simulink model "IQRD_RLS_model_top_3x3"  (R2020b)
settings: Solver=VariableStepAuto  StartTime=0.0  StopTime=0.00001  RelTol=1e-3
settings Model: Creator=jgentile  LastModifiedBy=jgentile

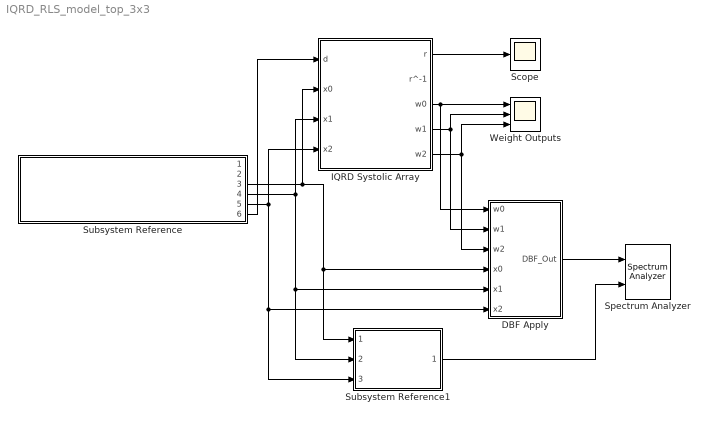
== system IQRD_RLS_model_top_3x3 ==
  DBF Apply : Subsystem
  IQRD Systolic Array : Subsystem
  Scope : Scope
  Spectrum Analyzer : SpectrumAnalyzer  NumInputPorts=2
  Subsystem Reference : Subsystem  ReferencedSubsystem=s3x3_ULA_additive_Noise_Interference
  Subsystem Reference1 : Subsystem  ReferencedSubsystem=Weighted_Sum_Avg_No_ABF
  Weight Outputs : Scope  NumInputPorts=3
  wires:
  IQRD Systolic Array/3(w0) -> Weight Outputs/1, DBF Apply/1(w0)
  IQRD Systolic Array/4(w1) -> Weight Outputs/2, DBF Apply/2(w1)
  IQRD Systolic Array/5(w2) -> Weight Outputs/3, DBF Apply/3(w2)
  Subsystem Reference/3 -> Subsystem Reference1/1, DBF Apply/4(x0), IQRD Systolic Array/2(x0)
  Subsystem Reference/4 -> Subsystem Reference1/2, DBF Apply/5(x1), IQRD Systolic Array/3(x1)
  Subsystem Reference/5 -> Subsystem Reference1/3, DBF Apply/6(x2), IQRD Systolic Array/4(x2)
  Subsystem Reference1/1 -> Spectrum Analyzer/2
  DBF Apply/1(DBF_Out) -> Spectrum Analyzer/1
  IQRD Systolic Array/1(r) -> Scope/1
  Subsystem Reference/6 -> IQRD Systolic Array/1(d)

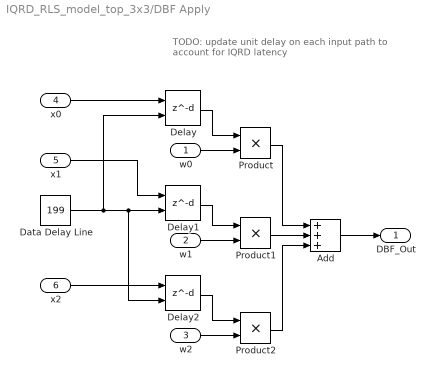
== system IQRD_RLS_model_top_3x3/DBF Apply ==
  note: TODO: update unit delay on each input path
      | to account for IQRD latency
  w0 : Inport
  w1 : Inport  Port=2
  w2 : Inport  Port=3
  x0 : Inport  Port=4
  x1 : Inport  Port=5
  x2 : Inport  Port=6
  Add : Sum  Inputs=+++
  Data Delay Line : Constant  Value=199
  Delay : Delay  DelayLengthSource=Input port
      settings: InputPortMap=u0,p1
  Delay1 : Delay  DelayLengthSource=Input port
      settings: InputPortMap=u0,p1
  Delay2 : Delay  DelayLengthSource=Input port
      settings: InputPortMap=u0,p1
  Product : Product
  Product1 : Product
  Product2 : Product
  DBF_Out : Outport
  wires:
  Data Delay Line/1 -> Delay1/2, Delay2/2, Delay/2
  Delay1/1 -> Product1/1
  Add/1 -> DBF_Out/1
  w0/1 -> Product/2
  Delay/1 -> Product/1
  Product/1 -> Add/1
  x1/1 -> Delay1/1
  x2/1 -> Delay2/1
  w1/1 -> Product1/2
  w2/1 -> Product2/2
  x0/1 -> Delay/1
  Delay2/1 -> Product2/1
  Product2/1 -> Add/3
  Product1/1 -> Add/2

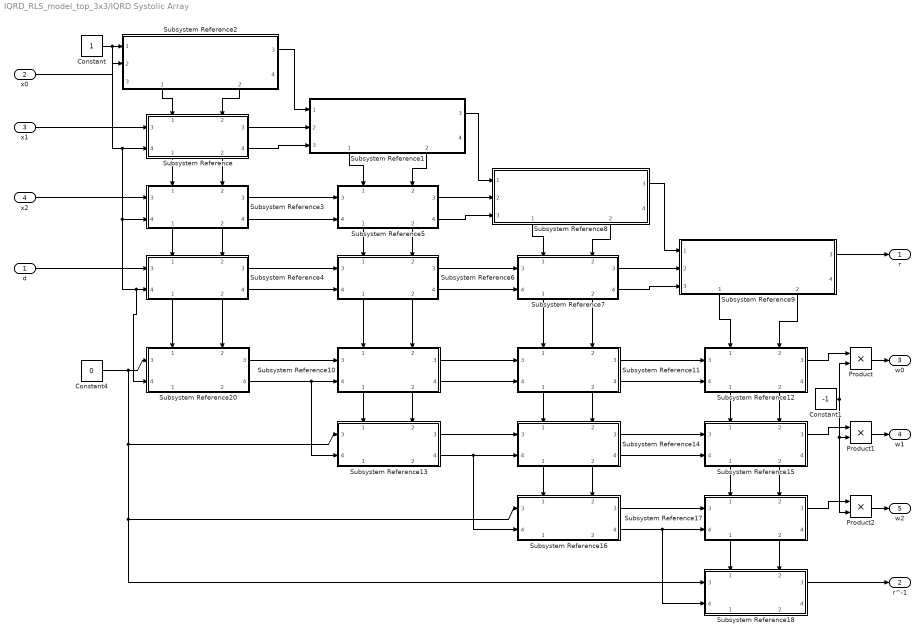
== system IQRD_RLS_model_top_3x3/IQRD Systolic Array ==
  d : Inport
  x0 : Inport  Port=2
  x1 : Inport  Port=3
  x2 : Inport  Port=4
  Constant : Constant
  Constant1 : Constant  Value=-1
  Constant4 : Constant  Value=0
  Product : Product
  Product1 : Product
  Product2 : Product
  Subsystem Reference{,3..7} (6 alike) : Subsystem  ReferencedSubsystem=internal_cell_givens
      settings: PortSchema="{\"entries\":[{\"content\":{\"sides\":[{\"content\":{\"connectorIds\":[\"In3\",\"In4\"]},\"type\":\"ConnectorPlacement.EquallySpacedRectSide\",\"uuid\":\"0239e4e7-44b6-4143-a587-38d4cded4ca6\"},{\"content\":{\"connectorIds\":[\"Out3\",\"Out4\"],\"side\":\"RIGHT\"},\"type\":\"ConnectorPlacement.EquallySpacedRectSide\",\"uuid\":\"ea23c866-1a25-41e9-a0f2-3862af1c86e1\"},{\"content\":{\"connectorIds\":[\"In1\",\"In2\"],\"side\":\"TOP\"},\"type\":\"ConnectorPlacement.EquallySpacedRectSide\",\"uuid\":\"8a8bb13e-2e16-40e7-9ca3-19d820578314\"},{\"content\":{\"connectorIds\":[\"Out1\",\"Out2\"],\"side\":\"BOTTOM\"},\"type\":\"ConnectorPlacement.EquallySpacedRectSide\",\"uuid\":\"1be66ea9-adc8-4a43-a798-b14d6fcab7cd\"},{\"content\":{\"connectorIds\":[],\"side\":\"HIDDEN\"},\"type\":\"ConnectorPlacement.EquallySpacedRectSide\",\"uuid\":\"0fecdaf4-55de-420b-b554-931c979049af\"}]},\"type\":\"ConnectorPlacement.EquallySpacedConnector\",\"uuid\":\"70182f79-db57-400d-a53f-39946a20555a\"}],\"packageUris\":[\"http://schema.mathworks.com/mf0/Connector/R2020b\"],\"version\":\"1.0\"}"
  Subsystem Reference{1..2,8..9} (4 alike) : Subsystem  ReferencedSubsystem=boundary_cell_givens
      settings: PortSchema="{\"entries\":[{\"content\":{\"sides\":[{\"content\":{\"connectorIds\":[\"In1\",\"In2\",\"In3\"]},\"type\":\"ConnectorPlacement.EquallySpacedRectSide\",\"uuid\":\"11c023aa-376d-416d-bfcd-8d7843f2be22\"},{\"content\":{\"connectorIds\":[\"Out3\",\"Out4\"],\"side\":\"RIGHT\"},\"type\":\"ConnectorPlacement.EquallySpacedRectSide\",\"uuid\":\"1a04016b-daba-4444-ad99-d7273a1feb5b\"},{\"content\":{\"connectorIds\":[],\"side\":\"TOP\"},\"type\":\"ConnectorPlacement.EquallySpacedRectSide\",\"uuid\":\"dd6dcf65-02b5-4ffa-b5ff-7e58c587941b\"},{\"content\":{\"connectorIds\":[\"Out1\",\"Out2\"],\"side\":\"BOTTOM\"},\"type\":\"ConnectorPlacement.EquallySpacedRectSide\",\"uuid\":\"26ecda3d-5bd8-4d7b-b858-e25b16c314b4\"},{\"content\":{\"connectorIds\":[],\"side\":\"HIDDEN\"},\"type\":\"ConnectorPlacement.EquallySpacedRectSide\",\"uuid\":\"bd7630cc-a9b8-4021-b6b5-0e32bd520d7d\"}]},\"type\":\"ConnectorPlacement.EquallySpacedConnector\",\"uuid\":\"7bb81265-b299-46b6-8c47-6bc2be69935c\"}],\"packageUris\":[\"http://schema.mathworks.com/mf0/Connector/R2020b\"],\"version\":\"1.0\"}"
  Subsystem Reference{10..18,20} (10 alike) : Subsystem  ReferencedSubsystem=inv_internal_cell_givens
      settings: PortSchema="{\"entries\":[{\"content\":{\"sides\":[{\"content\":{\"connectorIds\":[\"In3\",\"In4\"]},\"type\":\"ConnectorPlacement.EquallySpacedRectSide\",\"uuid\":\"7a30fd97-238e-4d3f-b86c-0b989816bca0\"},{\"content\":{\"connectorIds\":[\"Out3\",\"Out4\"],\"side\":\"RIGHT\"},\"type\":\"ConnectorPlacement.EquallySpacedRectSide\",\"uuid\":\"97592077-7dd1-4e2a-9ce3-178c2c88f4d0\"},{\"content\":{\"connectorIds\":[\"In1\",\"In2\"],\"side\":\"TOP\"},\"type\":\"ConnectorPlacement.EquallySpacedRectSide\",\"uuid\":\"6aed6abb-33ac-4a40-86f4-2f1f080d5792\"},{\"content\":{\"connectorIds\":[\"Out1\",\"Out2\"],\"side\":\"BOTTOM\"},\"type\":\"ConnectorPlacement.EquallySpacedRectSide\",\"uuid\":\"d6ad6c95-90c4-469b-9aab-57bb42a059b1\"},{\"content\":{\"connectorIds\":[],\"side\":\"HIDDEN\"},\"type\":\"ConnectorPlacement.EquallySpacedRectSide\",\"uuid\":\"5567bba2-9935-40d2-a99a-4fbdd449a1bc\"}]},\"type\":\"ConnectorPlacement.EquallySpacedConnector\",\"uuid\":\"249ba23d-f701-4623-a398-9ae5c4f4b120\"}],\"packageUris\":[\"http://schema.mathworks.com/mf0/Connector/R2020b\"],\"version\":\"1.0\"}"
  r : Outport
  r^-1 : Outport  Port=2
  w0 : Outport  Port=3
  w1 : Outport  Port=4
  w2 : Outport  Port=5
  wires:
  Subsystem Reference2/1 -> Subsystem Reference/1
  Subsystem Reference1/1 -> Subsystem Reference5/1
  Subsystem Reference3/3 -> Subsystem Reference5/3
  Subsystem Reference18/3 -> r^-1/1
  Subsystem Reference/3 -> Subsystem Reference1/2
  Subsystem Reference4/3 -> Subsystem Reference6/3
  Subsystem Reference6/3 -> Subsystem Reference7/3
  x0/1 -> Subsystem Reference2/2
  Subsystem Reference5/3 -> Subsystem Reference8/2
  Subsystem Reference3/2 -> Subsystem Reference4/2
  Subsystem Reference2/3 -> Subsystem Reference1/1
  Subsystem Reference/1 -> Subsystem Reference3/1
  Subsystem Reference7/3 -> Subsystem Reference9/2
  Subsystem Reference3/1 -> Subsystem Reference4/1
  Subsystem Reference/2 -> Subsystem Reference3/2
  Constant/1 -> Subsystem Reference20/4, Subsystem Reference4/4, Subsystem Reference3/4, Subsystem Reference/4, Subsystem Reference2/1
  Subsystem Reference1/3 -> Subsystem Reference8/1
  Subsystem Reference5/2 -> Subsystem Reference6/2
  Subsystem Reference5/1 -> Subsystem Reference6/1
  Subsystem Reference2/2 -> Subsystem Reference/2
  Subsystem Reference8/3 -> Subsystem Reference9/1
  Subsystem Reference8/2 -> Subsystem Reference7/2
  Subsystem Reference1/2 -> Subsystem Reference5/2
  Subsystem Reference8/1 -> Subsystem Reference7/1
  Constant4/1 -> Subsystem Reference13/3, Subsystem Reference18/3, Subsystem Reference16/3, Subsystem Reference20/3
  Subsystem Reference4/1 -> Subsystem Reference20/1
  Subsystem Reference4/2 -> Subsystem Reference20/2
  Subsystem Reference6/1 -> Subsystem Reference10/1
  Subsystem Reference6/2 -> Subsystem Reference10/2
  Subsystem Reference7/1 -> Subsystem Reference11/1
  Subsystem Reference7/2 -> Subsystem Reference11/2
  Subsystem Reference9/1 -> Subsystem Reference12/1
  Subsystem Reference9/2 -> Subsystem Reference12/2
  Subsystem Reference20/3 -> Subsystem Reference10/3
  Subsystem Reference10/3 -> Subsystem Reference11/3
  Subsystem Reference11/3 -> Subsystem Reference12/3
  Subsystem Reference10/1 -> Subsystem Reference13/1
  Subsystem Reference10/2 -> Subsystem Reference13/2
  Subsystem Reference11/1 -> Subsystem Reference14/1
  Subsystem Reference11/2 -> Subsystem Reference14/2
  Subsystem Reference12/1 -> Subsystem Reference15/1
  Subsystem Reference12/2 -> Subsystem Reference15/2
  Subsystem Reference14/1 -> Subsystem Reference16/1
  Subsystem Reference14/2 -> Subsystem Reference16/2
  Subsystem Reference15/1 -> Subsystem Reference17/1
  Subsystem Reference15/2 -> Subsystem Reference17/2
  Subsystem Reference17/1 -> Subsystem Reference18/1
  Subsystem Reference17/2 -> Subsystem Reference18/2
  Subsystem Reference13/3 -> Subsystem Reference14/3
  Subsystem Reference14/3 -> Subsystem Reference15/3
  Subsystem Reference16/3 -> Subsystem Reference17/3
  x1/1 -> Subsystem Reference/3
  x2/1 -> Subsystem Reference3/3
  d/1 -> Subsystem Reference4/3
  Subsystem Reference9/3 -> r/1
  Subsystem Reference/4 -> Subsystem Reference1/3
  Subsystem Reference3/4 -> Subsystem Reference5/4
  Subsystem Reference4/4 -> Subsystem Reference6/4
  Subsystem Reference20/4 -> Subsystem Reference10/4, Subsystem Reference13/4
  Subsystem Reference5/4 -> Subsystem Reference8/3
  Subsystem Reference6/4 -> Subsystem Reference7/4
  Subsystem Reference10/4 -> Subsystem Reference11/4
  Subsystem Reference13/4 -> Subsystem Reference16/4, Subsystem Reference14/4
  Subsystem Reference7/4 -> Subsystem Reference9/3
  Subsystem Reference11/4 -> Subsystem Reference12/4
  Subsystem Reference14/4 -> Subsystem Reference15/4
  Subsystem Reference16/4 -> Subsystem Reference18/4, Subsystem Reference17/4
  Product/1 -> w0/1
  Product1/1 -> w1/1
  Product2/1 -> w2/1
  Subsystem Reference12/3 -> Product/1
  Subsystem Reference15/3 -> Product1/1
  Subsystem Reference17/3 -> Product2/1
  Constant1/1 -> Product2/2, Product1/2, Product/2
